simulink model "test"  (R2017a)
settings: Solver=VariableStepAuto  StartTime=0.0  StopTime=10.0  RelTol=1e-3
values from neighbouring files (symbols this model uses):
  b = 2    [test_mfile.m]
  c = 3    [test_mfile.m]
  F = 10    [test_mfile.m]
  m = 2000    [Tire_dugoff_part2.m]    (also in Tire_dugoff_starter.m; test_mfile.m = 5)
settings Model: Creator=Instructor  LastModifiedBy=Instructor

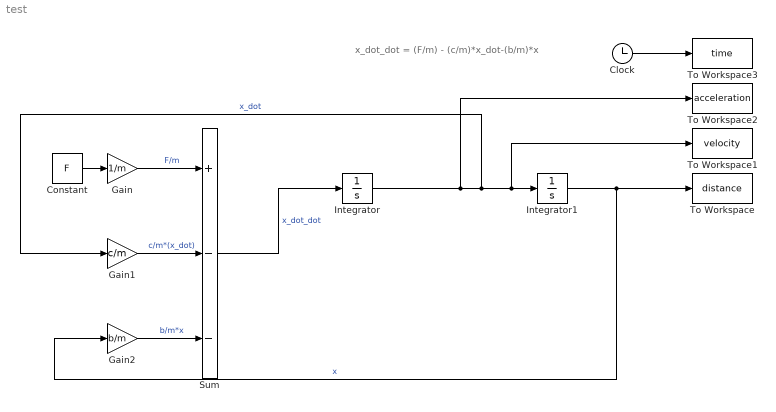
== system test ==
  note: x_dot_dot = (F/m) - (c/m)*x_dot-(b/m)*x
  Clock : Clock
  Constant : Constant  Value=F
  Gain : Gain  Gain=1/m
  Gain1 : Gain  Gain=c/m
  Gain2 : Gain  Gain=b/m
  Integrator : Integrator  InitialCondition=5
  Integrator1 : Integrator
  Sum : Sum  Inputs=+--
  To Workspace : ToWorkspace  VariableName=distance  SampleTime=-1
  To Workspace1 : ToWorkspace  VariableName=velocity  SampleTime=-1
  To Workspace2 : ToWorkspace  VariableName=acceleration  SampleTime=-1
  To Workspace3 : ToWorkspace  VariableName=time  SampleTime=-1
  wires:
  Integrator/1 -> To Workspace2/1, Gain1/1, To Workspace1/1, Integrator1/1  "x_dot"
  Sum/1 -> Integrator/1  "x_dot_dot"
  Integrator1/1 -> To Workspace/1, Gain2/1  "x"
  Constant/1 -> Gain/1
  Gain/1 -> Sum/1  "F/m"
  Gain1/1 -> Sum/2  "c/m*(x_dot)"
  Gain2/1 -> Sum/3  "b/m*x"
  Clock/1 -> To Workspace3/1
